simulink model "Powertrain_model_BE_21a"  (R2021a)
settings: Solver=VariableStepAuto  StartTime=0.0  StopTime=10800  RelTol=1e-3
values from neighbouring files (symbols this model uses):
  DR = 5.213    [Sim_script.m]    (also in workspace.mat)
  eta_EM_map = [0.5831 0.6831 0.781 0.826 0 0 0 0 0 0.6107 0.7107 0.8049 ... (270 elements, 9x30)]    [workspace.mat]
  Gensetdata = Gensetdata2    [Sim_script.m]    (also in fuel_con_map_Sagar.m = [0	    268.270328038217)
  rated_pow_M = 2002    [Sim_script.m]    (also in workspace.mat)
  T_EM_col = [-74.73 -59.49 -53.55 -49.77 -44.93 -40 -34.96 -30.36 -25.1 -20.31 -15.68 -10.18 ... (30 elements, 30x1)]    [workspace.mat]
  T_EM_max = [70 70 70 52 38 28 19 13 9]    [workspace.mat]
  Trans_In = 24.086    [Sim_script.m]    (also in workspace.mat)
  w_CE_idle = 400    [Sim_script.m]    (also in workspace.mat = 32)
  w_EM_row = [0 75 150 225 300 375 450 525 600]    [workspace.mat]
undefined symbols (not defined in the file or in its folder): dailyloadl, induction_lookup, motor_eff_IND, resT
libraries: pid_lib x1
settings Model: Creator=user  LastModifiedBy=olsonsao

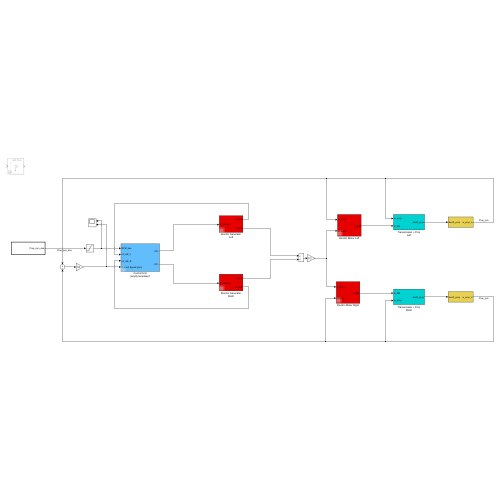
[thumbnail: Simulink's stored preview of the top-level diagram]
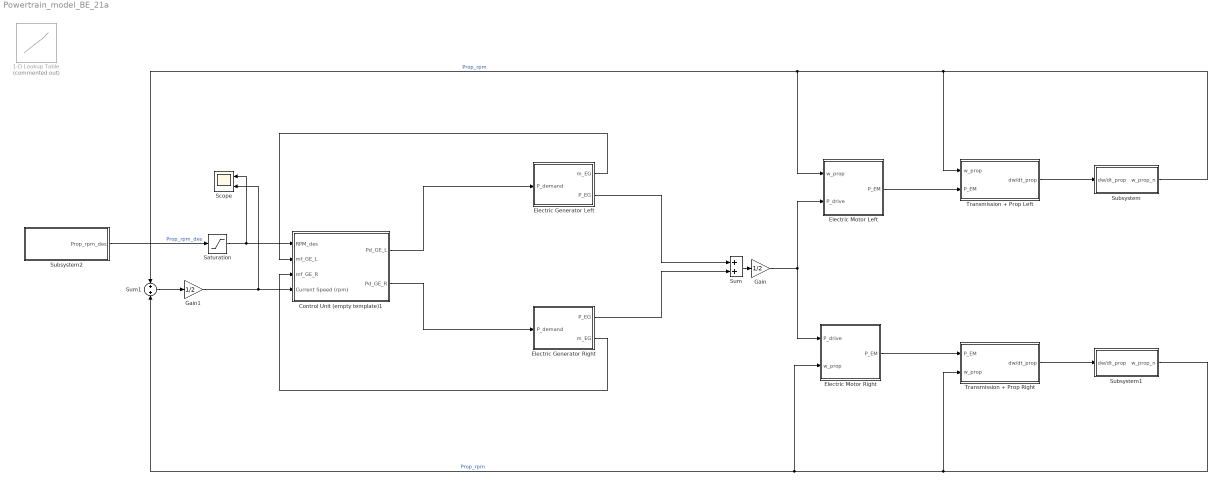
== system Powertrain_model_BE_21a ==
  1-D Lookup Table : Lookup_n-D  Commented=on  NumberOfTableDimensions=1  BreakpointsForDimension1=power  Table=induction_lookup  InternalRulePriority=Speed  RndMeth=Simplest  InputSameDT=on
  Control Unit (empty template)1 : Subsystem  Tag=control unit  AncestorBlock=|
      | qss_tb_library/Controller/Control Unit
      | (empty template)
  Electric Generator Left : Subsystem  AncestorBlock=qss_tb_library/Energy Converter/Electric Generator
  Electric Generator Right : Subsystem  AncestorBlock=qss_tb_library/Energy Converter/Electric Generator
  Electric Motor Left : Subsystem  AncestorBlock=qss_tb_library/Energy Converter/Electric Motor
  Electric Motor Right : Subsystem  AncestorBlock=qss_tb_library/Energy Converter/Electric Motor
  Gain : Gain  Gain=1/2
  Gain1 : Gain  Gain=1/2
  Saturation : Saturate  UpperLimit=inf  LowerLimit=w_CE_idle
  Scope : Scope  NumInputPorts=2
  Subsystem : Subsystem
  Subsystem1 : Subsystem
  Subsystem2 : Subsystem  TreatAsAtomicUnit=on
  Sum : Sum
  Sum1 : Sum  Inputs=+|+
  Transmission + Prop Left : Subsystem
  Transmission + Prop Right : Subsystem
  wires:
  Sum/1 -> Gain/1
  Gain/1 -> Electric Motor Left/2(P_drive), Electric Motor Right/1(P_drive)
  Electric Motor Left/1(P_EM) -> Transmission + Prop Left/2(P_EM)
  Subsystem/1(w_prop_n) -> Transmission + Prop Left/1(w_prop), Sum1/1, Electric Motor Left/1(w_prop)  "Prop_rpm"
  Control Unit (empty template)1/1(Pd_GE_L) -> Electric Generator Left/1(P_demand)
  Electric Motor Right/1(P_EM) -> Transmission + Prop Right/1(P_EM)
  Subsystem1/1(w_prop_n) -> Sum1/2, Electric Motor Right/2(w_prop), Transmission + Prop Right/2(w_prop)  "Prop_rpm"
  Control Unit (empty template)1/2(Pd_GE_R) -> Electric Generator Right/1(P_demand)
  Gain1/1 -> Scope/2, Control Unit (empty template)1/4(Current Speed (rpm))
  Subsystem2/1(Prop_rpm_des) -> Saturation/1  "Prop_rpm_des"
  Saturation/1 -> Scope/1, Control Unit (empty template)1/1(RPM_des)
  Electric Generator Left/2(P_EG) -> Sum/1
  Electric Generator Left/1(m_EG) -> Control Unit (empty template)1/2(mf_GE_L)
  Electric Generator Right/1(P_EG) -> Sum/2
  Electric Generator Right/2(m_EG) -> Control Unit (empty template)1/3(mf_GE_R)
  Sum1/1 -> Gain1/1
  Transmission + Prop Left/1(dw/dt_prop) -> Subsystem/1(dw/dt_prop)
  Transmission + Prop Right/1(dw/dt_prop) -> Subsystem1/1(dw/dt_prop)

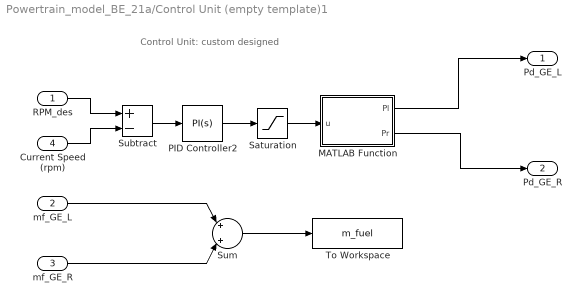
== system Powertrain_model_BE_21a/Control Unit (empty template)1 ==
  note: Control Unit: custom designed
  RPM_des : Inport
  mf_GE_L : Inport  Port=2
  mf_GE_R : Inport  Port=3
  Current Speed (rpm) : Inport  Port=4
  MATLAB Function : MATLAB Function  TreatAsAtomicUnit=on
  PID Controller2 : pid_lib/PID Controller  Controller=PI  Form=Parallel  TimeDomain=Continuous-time  UseExternalTs=off  SampleTime=-1  IntegratorMethod=Forward Euler  FilterMethod=Forward Euler  ControllerParametersSource=internal  P=0.408569070042623  I=0.0614231998604096  D=0.13961986597848  UseFilter=on  N=2.64189049403583  TunerSelectOption=Transfer Function Based (PID Tuner App)  InitialConditionSource=internal  InitialConditionForIntegrator=0  InitialConditionForFilter=0  DifferentiatorICPrevScaledInput=0  ExternalReset=none  TrackingMode=off  Kt=1  LimitOutput=on  SatLimitsSource=internal  UpperSaturationLimit=inf  LowerSaturationLimit=0  LinearizeAsGain=off  AntiWindupMode=none  Kb=1  POutMin=[]  POutMax=[]  IOutMin=[]  IOutMax=[]  DOutMin=[]  DOutMax=[]  NOutMin=[]  NOutMax=[]  SumOutMin=[]  SumOutMax=[]  SaturationOutMin=[]  SaturationOutMax=[]  PParamMin=[]  PParamMax=[]  IParamMin=[]  IParamMax=[]  DParamMin=[]  DParamMax=[]  NParamMin=[]  NParamMax=[]  KbParamMin=[]  KbParamMax=[]  KtParamMin=[]  KtParamMax=[]  KbOutMin=[]  KbOutMax=[]  KtOutMin=[]  KtOutMax=[]  IntegratorOutMin=[]  IntegratorOutMax=[]  FilterOutMin=[]  FilterOutMax=[]  SumI1OutMin=[]  SumI1OutMax=[]  SumI2OutMin=[]  SumI2OutMax=[]  SumI3OutMin=[]  SumI3OutMax=[]  SumI4OutMin=[]  SumI4OutMax=[]  SumDOutMin=[]  SumDOutMax=[]  DifferentiatorOutMin=[]  DifferentiatorOutMax=[]  FilterDiffOutCoefMin=[]  FilterDiffOutCoefMax=[]  ReciprocalOutMin=[]  ReciprocalOutMax=[]  SumDenOutMin=[]  SumDenOutMax=[]  SumNumOutMin=[]  SumNumOutMax=[]  DivideOutMin=[]  DivideOutMax=[]  UdiffTsProdOutMin=[]  UdiffTsProdOutMax=[]  NTsProdOutMin=[]  NTsProdOutMax=[]  UintegralTsProdOutMin=[]  UintegralTsProdOutMax=[]  UngainTsProdOutMin=[]  UngainTsProdOutMax=[]  IntegratorContinuousStateAttributes=''  IntegratorStateMustResolveToSignalObject=off  IntegratorRTWStateStorageClass=Auto  FilterContinuousStateAttributes=''  FilterStateMustResolveToSignalObject=off  FilterRTWStateStorageClass=Auto  ParallelPVariant=InternalParameters  IdealPVariant=Disabled  IVariant=InternalParameters  DVariant=Disabled  IntegratorVariant=Continuous  SatVariant=Enabled  AWVariant=Passthrough  PCopyVariant=Disabled  TRVariant=Disabled  FdbkBlocksVariant=Forward  IdealPFdbkVariant=Disabled  SatFdbkVariant=Disabled  DerivativeFilterVariant=Disabled  NVariant=Disabled  NCopyVariant=Disabled_SignalSpec  FilterICVariant=Disabled  IntegratorICVariant=InternalICs  ExternalResetVariant=Disabled  TRSumVariant=Passthrough  SumFdbkVariant=Disabled  SumVariant=Sum_PI  TsampFilterVariant=InternalTs  TsampNgainVariant=Passthrough  TsampIntegralVariant=Passthrough  ExternalSaturationOutDataTypeStr=Inherit: Same as second input
  Saturation : Saturate  UpperLimit=4172  LowerLimit=0
  Subtract : Sum  Inputs=+-
  Sum : Sum  Inputs=|+|+|
  To Workspace : ToWorkspace  VariableName=m_fuel  SampleTime=-1
      settings: Save2DSignal=2-D array (concatenate along first dimension)
  Pd_GE_L : Outport  InitialOutput=0
  Pd_GE_R : Outport  Port=2  InitialOutput=0
  wires:
  Current Speed (rpm)/1 -> Subtract/2
  RPM_des/1 -> Subtract/1
  Subtract/1 -> PID Controller2/1
  mf_GE_L/1 -> Sum/1
  mf_GE_R/1 -> Sum/2
  PID Controller2/1 -> Saturation/1
  Saturation/1 -> MATLAB Function/1(u)
  Sum/1 -> To Workspace/1
  MATLAB Function/2(Pr) -> Pd_GE_R/1
  MATLAB Function/1(Pl) -> Pd_GE_L/1

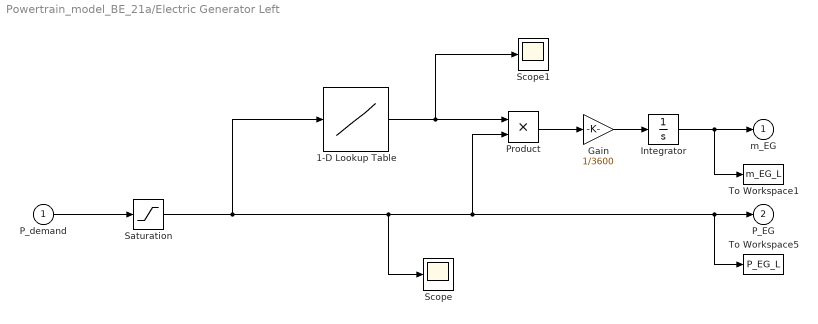
== system Powertrain_model_BE_21a/Electric Generator Left ==
  P_demand : Inport
  1-D Lookup Table : Lookup_n-D  NumberOfTableDimensions=1  BreakpointsForDimension1=Gensetdata.('Power(kW)')  Table=Gensetdata.('Bsfc(g/kWh)')  InterpMethod=Cubic spline  ExtrapMethod=Cubic spline  InternalRulePriority=Speed  RndMeth=Simplest  InputSameDT=on
  Gain : Gain  Gain=1/3600
  Integrator : Integrator
  Product : Product
  Saturation : Saturate  UpperLimit=2500  LowerLimit=0
  Scope : Scope
  Scope1 : Scope
  To Workspace1 : ToWorkspace  VariableName=m_EG_L  SampleTime=-1
      settings: Save2DSignal=2-D array (concatenate along first dimension)
  To Workspace5 : ToWorkspace  VariableName=P_EG_L  SampleTime=-1
      settings: Save2DSignal=2-D array (concatenate along first dimension)
  m_EG : Outport  InitialOutput=0
  P_EG : Outport  Port=2  InitialOutput=0
  wires:
  Integrator/1 -> m_EG/1, To Workspace1/1
  Gain/1 -> Integrator/1
  Product/1 -> Gain/1
  1-D Lookup Table/1 -> Scope1/1, Product/1
  P_demand/1 -> Saturation/1
  Saturation/1 -> Scope/1, P_EG/1, To Workspace5/1, Product/2, 1-D Lookup Table/1

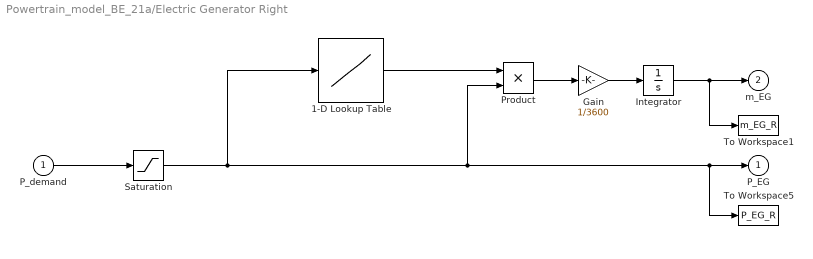
== system Powertrain_model_BE_21a/Electric Generator Right ==
  P_demand : Inport
  1-D Lookup Table : Lookup_n-D  NumberOfTableDimensions=1  BreakpointsForDimension1=Gensetdata.('Power(kW)')  Table=Gensetdata.('Bsfc(g/kWh)')  InterpMethod=Cubic spline  ExtrapMethod=Cubic spline  InternalRulePriority=Speed  RndMeth=Simplest  InputSameDT=on
  Gain : Gain  Gain=1/3600
  Integrator : Integrator
  Product : Product
  Saturation : Saturate  UpperLimit=2500  LowerLimit=0
  To Workspace1 : ToWorkspace  VariableName=m_EG_R  SampleTime=-1
      settings: Save2DSignal=2-D array (concatenate along first dimension)
  To Workspace5 : ToWorkspace  VariableName=P_EG_R  SampleTime=-1
      settings: Save2DSignal=2-D array (concatenate along first dimension)
  P_EG : Outport  InitialOutput=0
  m_EG : Outport  Port=2  InitialOutput=0
  wires:
  Integrator/1 -> m_EG/1, To Workspace1/1
  Gain/1 -> Integrator/1
  Product/1 -> Gain/1
  1-D Lookup Table/1 -> Product/1
  P_demand/1 -> Saturation/1
  Saturation/1 -> P_EG/1, To Workspace5/1, Product/2, 1-D Lookup Table/1

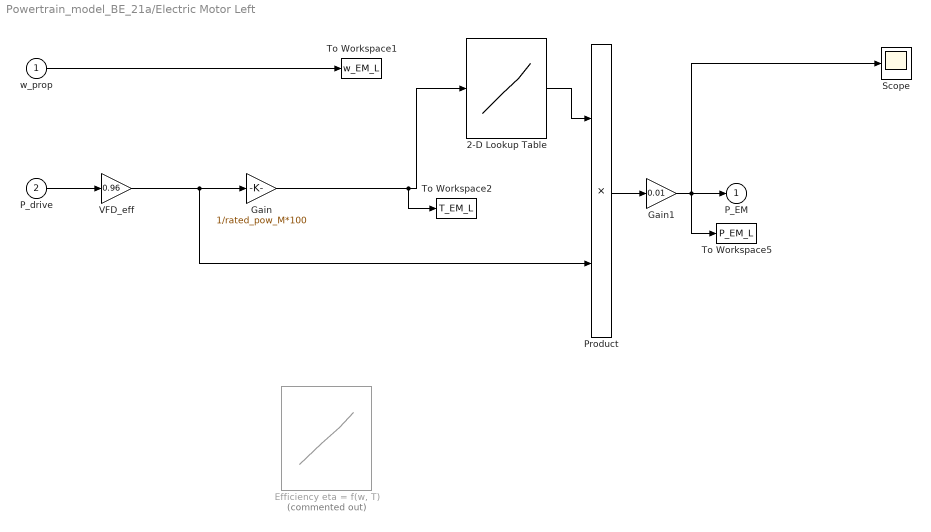
== system Powertrain_model_BE_21a/Electric Motor Left ==
  w_prop : Inport
  P_drive : Inport  Port=2
  2-D Lookup Table : Lookup_n-D  NumberOfTableDimensions=1  BreakpointsForDimension1=motor_eff_IND.('%power')  BreakpointsForDimension2=T_EM_col  Table=motor_eff_IND.('eff')  InterpMethod=Cubic spline  ExtrapMethod=Cubic spline  InternalRulePriority=Speed  RndMeth=Simplest  InputSameDT=on
  "Efficiency eta = f(w, T)" : Lookup2D  Commented=on  RowIndex=w_EM_row  ColumnIndex=T_EM_col  Table=eta_EM_map
  Gain : Gain  Gain=1/rated_pow_M*100
  Gain1 : Gain  Gain=0.01
  Product : Product  InputSameDT=on  RndMeth=Zero  SaturateOnIntegerOverflow=on  OutDataTypeStr=Inherit: Same as first input
  Scope : Scope
  To Workspace1 : ToWorkspace  VariableName=w_EM_L  SampleTime=-1
      settings: Save2DSignal=2-D array (concatenate along first dimension)
  To Workspace2 : ToWorkspace  VariableName=T_EM_L  SampleTime=-1
      settings: Save2DSignal=2-D array (concatenate along first dimension)
  To Workspace5 : ToWorkspace  VariableName=P_EM_L  SampleTime=-1
      settings: Save2DSignal=2-D array (concatenate along first dimension)
  VFD_eff : Gain  Gain=0.96
  P_EM : Outport  InitialOutput=0
  wires:
  Product/1 -> Gain1/1
  P_drive/1 -> VFD_eff/1
  2-D Lookup Table/1 -> Product/1
  w_prop/1 -> To Workspace1/1
  Gain/1 -> To Workspace2/1, 2-D Lookup Table/1
  VFD_eff/1 -> Gain/1, Product/2
  Gain1/1 -> Scope/1, To Workspace5/1, P_EM/1

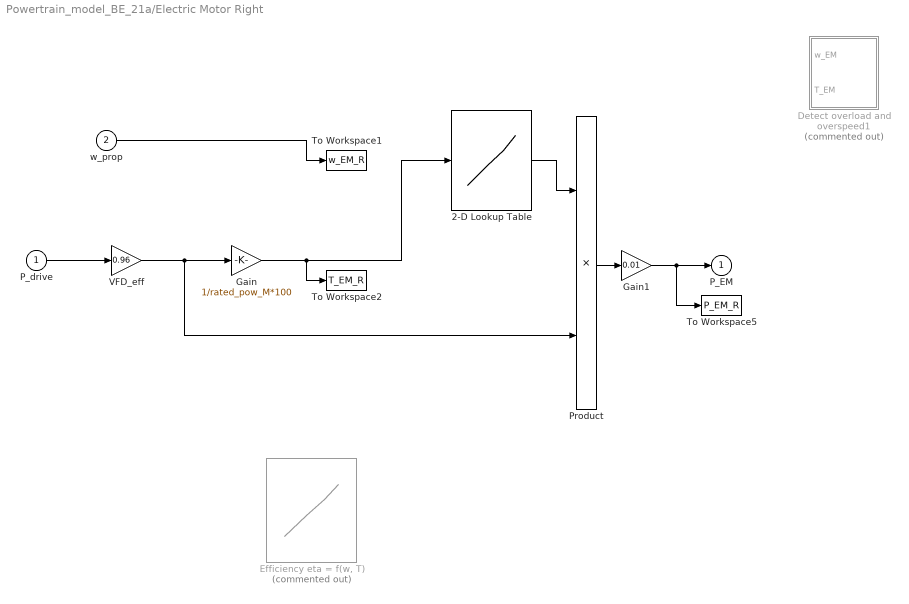
== system Powertrain_model_BE_21a/Electric Motor Right ==
  P_drive : Inport
  w_prop : Inport  Port=2
  2-D Lookup Table : Lookup_n-D  NumberOfTableDimensions=1  BreakpointsForDimension1=motor_eff_IND.('%power')  BreakpointsForDimension2=T_EM_col  Table=motor_eff_IND.('eff')  InterpMethod=Cubic spline  ExtrapMethod=Cubic spline  InternalRulePriority=Speed  RndMeth=Simplest  InputSameDT=on
  Detect overload and overspeed1 : Subsystem  Commented=on
  "Efficiency eta = f(w, T)" : Lookup2D  Commented=on  RowIndex=w_EM_row  ColumnIndex=T_EM_col  Table=eta_EM_map
  Gain : Gain  Gain=1/rated_pow_M*100
  Gain1 : Gain  Gain=0.01
  Product : Product  InputSameDT=on  RndMeth=Zero  SaturateOnIntegerOverflow=on  OutDataTypeStr=Inherit: Same as first input
  To Workspace1 : ToWorkspace  VariableName=w_EM_R  SampleTime=-1
      settings: Save2DSignal=2-D array (concatenate along first dimension)
  To Workspace2 : ToWorkspace  VariableName=T_EM_R  SampleTime=-1
      settings: Save2DSignal=2-D array (concatenate along first dimension)
  To Workspace5 : ToWorkspace  VariableName=P_EM_R  SampleTime=-1
      settings: Save2DSignal=2-D array (concatenate along first dimension)
  VFD_eff : Gain  Gain=0.96
  P_EM : Outport  InitialOutput=0
  wires:
  Product/1 -> Gain1/1
  P_drive/1 -> VFD_eff/1
  2-D Lookup Table/1 -> Product/1
  w_prop/1 -> To Workspace1/1
  Gain/1 -> To Workspace2/1, 2-D Lookup Table/1
  VFD_eff/1 -> Gain/1, Product/2
  Gain1/1 -> To Workspace5/1, P_EM/1

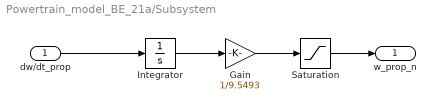
== system Powertrain_model_BE_21a/Subsystem ==
  dw/dt_prop : Inport
  Gain : Gain  Gain=1/9.5493
  Integrator : Integrator  InitialCondition=w_CE_idle
  Saturation : Saturate  UpperLimit=inf  LowerLimit=w_CE_idle
  w_prop_n : Outport
  wires:
  dw/dt_prop/1 -> Integrator/1
  Integrator/1 -> Gain/1
  Saturation/1 -> w_prop_n/1
  Gain/1 -> Saturation/1

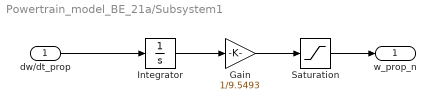
== system Powertrain_model_BE_21a/Subsystem1 ==
  dw/dt_prop : Inport
  Gain : Gain  Gain=1/9.5493
  Integrator : Integrator  InitialCondition=w_CE_idle
  Saturation : Saturate  UpperLimit=inf  LowerLimit=w_CE_idle
  w_prop_n : Outport
  wires:
  dw/dt_prop/1 -> Integrator/1
  Integrator/1 -> Gain/1
  Saturation/1 -> w_prop_n/1
  Gain/1 -> Saturation/1

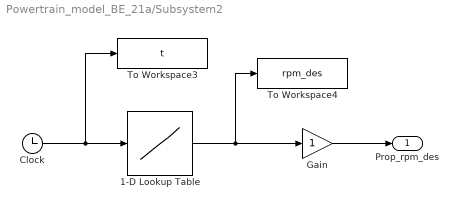
== system Powertrain_model_BE_21a/Subsystem2 ==
  1-D Lookup Table : Lookup_n-D  NumberOfTableDimensions=1  BreakpointsForDimension1=[1:10800]  Table=dailyloadl.('m_sec')  InternalRulePriority=Speed  RndMeth=Simplest  InputSameDT=on
  Clock : Clock
  Gain : Gain
  To Workspace3 : ToWorkspace  VariableName=t  SampleTime=-1
      settings: Save2DSignal=2-D array (concatenate along first dimension)
  To Workspace4 : ToWorkspace  VariableName=rpm_des  SampleTime=-1
      settings: Save2DSignal=2-D array (concatenate along first dimension)
  Prop_rpm_des : Outport
  wires:
  Clock/1 -> To Workspace3/1, 1-D Lookup Table/1
  1-D Lookup Table/1 -> Gain/1, To Workspace4/1
  Gain/1 -> Prop_rpm_des/1

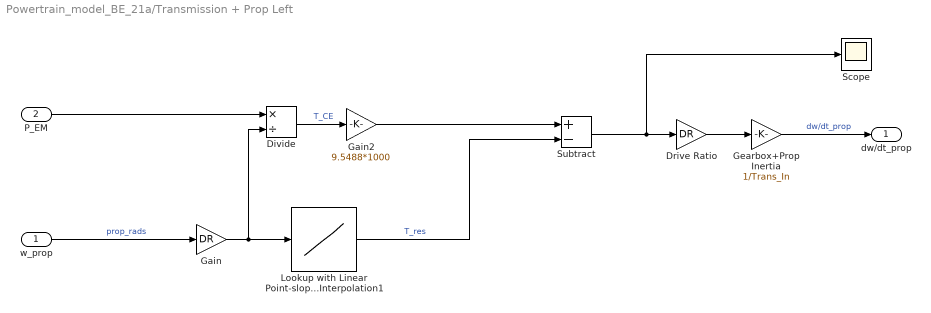
== system Powertrain_model_BE_21a/Transmission + Prop Left ==
  w_prop : Inport
  P_EM : Inport  Port=2
  Divide : Product  Inputs=*/
  Drive Ratio : Gain  Gain=DR
  Gain : Gain  Gain=DR
  Gain2 : Gain  Gain=9.5488*1000
  Gearbox+Prop Inertia : Gain  Gain=1/Trans_In
  Lookup with Linear Point-slope Interpolation1 : Lookup_n-D  NumberOfTableDimensions=1  BreakpointsForDimension1=resT.('rpm')  Table=resT.('resT')  InternalRulePriority=Speed  RndMeth=Simplest  InputSameDT=on
  Scope : Scope
  Subtract : Sum  Inputs=+-
  dw/dt_prop : Outport
  wires:
  Lookup with Linear Point-slope Interpolation1/1 -> Subtract/2  "T_res"
  P_EM/1 -> Divide/1
  Subtract/1 -> Scope/1, Drive Ratio/1
  Gearbox+Prop Inertia/1 -> dw/dt_prop/1  "dw/dt_prop"
  Drive Ratio/1 -> Gearbox+Prop Inertia/1
  Divide/1 -> Gain2/1  "T_CE"
  Gain/1 -> Lookup with Linear Point-slope Interpolation1/1, Divide/2
  Gain2/1 -> Subtract/1
  w_prop/1 -> Gain/1  "prop_rads"

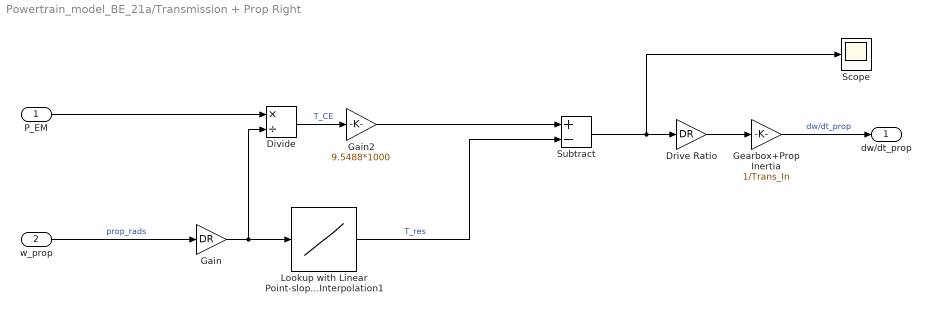
== system Powertrain_model_BE_21a/Transmission + Prop Right ==
  P_EM : Inport
  w_prop : Inport  Port=2
  Divide : Product  Inputs=*/
  Drive Ratio : Gain  Gain=DR
  Gain : Gain  Gain=DR
  Gain2 : Gain  Gain=9.5488*1000
  Gearbox+Prop Inertia : Gain  Gain=1/Trans_In
  Lookup with Linear Point-slope Interpolation1 : Lookup_n-D  NumberOfTableDimensions=1  BreakpointsForDimension1=resT.('rpm')  Table=resT.('resT')  InternalRulePriority=Speed  RndMeth=Simplest  InputSameDT=on
  Scope : Scope
  Subtract : Sum  Inputs=+-
  dw/dt_prop : Outport
  wires:
  Lookup with Linear Point-slope Interpolation1/1 -> Subtract/2  "T_res"
  P_EM/1 -> Divide/1
  Subtract/1 -> Scope/1, Drive Ratio/1
  Gearbox+Prop Inertia/1 -> dw/dt_prop/1  "dw/dt_prop"
  Drive Ratio/1 -> Gearbox+Prop Inertia/1
  Divide/1 -> Gain2/1  "T_CE"
  Gain/1 -> Lookup with Linear Point-slope Interpolation1/1, Divide/2
  Gain2/1 -> Subtract/1
  w_prop/1 -> Gain/1  "prop_rads"

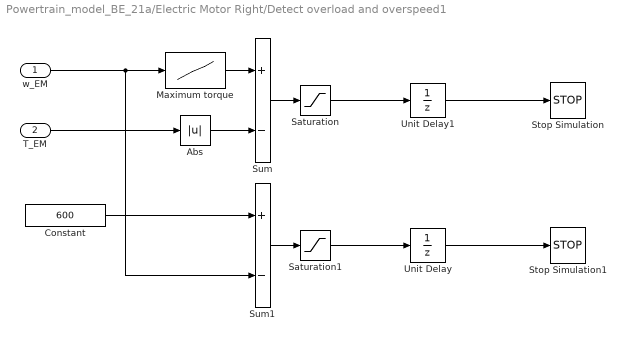
== system Powertrain_model_BE_21a/Electric Motor Right/Detect overload and overspeed1 ==
  w_EM : Inport
  T_EM : Inport  Port=2
  Abs : Abs  SaturateOnIntegerOverflow=on
  Constant : Constant  Value=600
  Maximum torque : Lookup  InputValues=w_EM_row  Table=T_EM_max  SaturateOnIntegerOverflow=on
  Saturation : Saturate  UpperLimit=0  LowerLimit=-inf
  Saturation1 : Saturate  UpperLimit=0  LowerLimit=-inf
  Stop Simulation : Stop
  Stop Simulation1 : Stop
  Sum : Sum  Inputs=+-  InputSameDT=on  SaturateOnIntegerOverflow=on  OutDataTypeStr=Inherit: Same as first input
  Sum1 : Sum  Inputs=+-  InputSameDT=on  SaturateOnIntegerOverflow=on  OutDataTypeStr=Inherit: Same as first input
  Unit Delay : UnitDelay  SampleTime=-1  HasFrameUpgradeWarning=on
  Unit Delay1 : UnitDelay  SampleTime=-1  HasFrameUpgradeWarning=on
  wires:
  Saturation1/1 -> Unit Delay/1
  Sum1/1 -> Saturation1/1
  Constant/1 -> Sum1/1
  Saturation/1 -> Unit Delay1/1
  Abs/1 -> Sum/2
  Maximum torque/1 -> Sum/1
  T_EM/1 -> Abs/1
  w_EM/1 -> Sum1/2, Maximum torque/1
  Sum/1 -> Saturation/1
  Unit Delay/1 -> Stop Simulation1/1
  Unit Delay1/1 -> Stop Simulation/1

== matlab function Powertrain_model_BE_21a/Control Unit (empty template)1/MATLAB Function ==
  data: u input; Pl output; Pr output
function [Pl,Pr] = fcn(u)

if u < 2500
    Pl = u;
    Pr = 0;
else
    Pl = 2500;
    Pr = u-2500;
end
end
